simulink model "advanced_control_simulink"  (R2025b)
settings: Solver=ode3  StartTime=0.0  StopTime=50  FixedStep=0.02  RelTol=1e-3
libraries: fuzblock x1
settings Model: Creator=Mohamed Zein  LastModifiedBy=Mohamed Zein

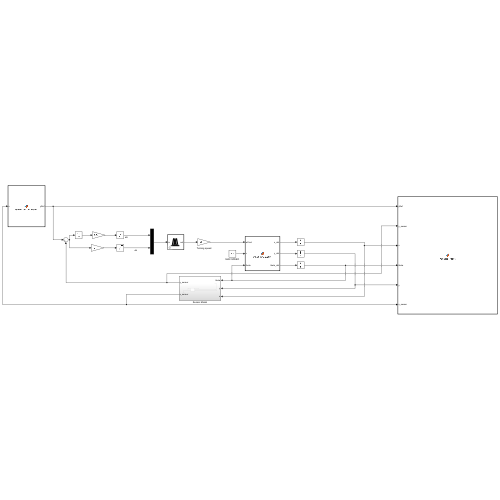
[thumbnail: Simulink's stored preview of the top-level diagram]
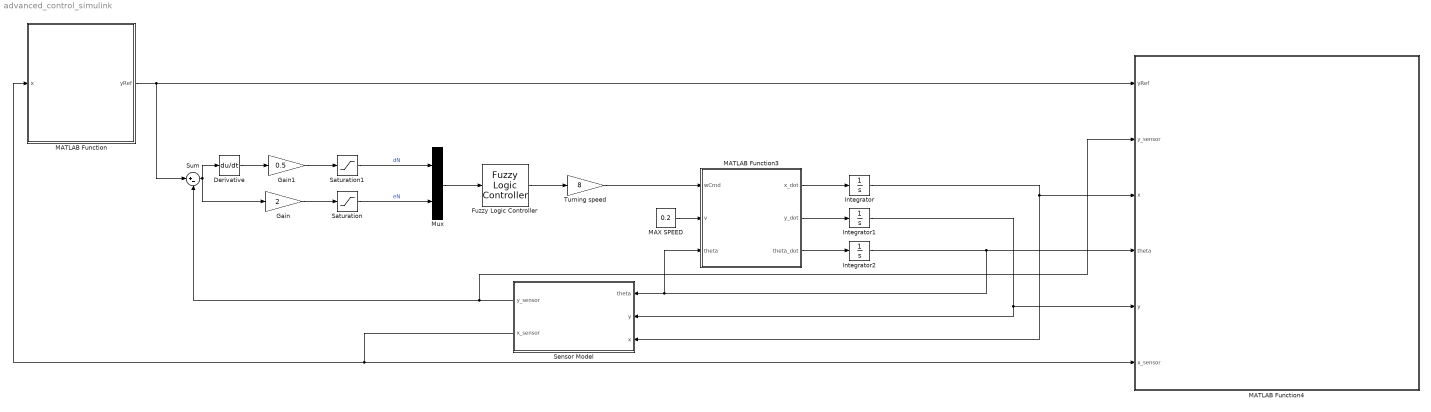
== system advanced_control_simulink ==
  Derivative : Derivative
  Fuzzy Logic Controller : fuzblock/Fuzzy Logic  Controller  FIS=fis  OutputSampleNumber=101  DataType=double  UseLookupTable=off  NumBreakpoints=10  FuzzifiedInputs=off  RuleFiringStrengths=off  RuleOutputs=off  AggregatedOutputs=off  SimulateUsing=Interpreted execution  OutOfRangeInputValueMessage=warning  NoRuleFiredMessage=warning  EmptyOutputFuzzySetMessage=warning
  Gain : Gain  Gain=2
  Gain1 : Gain  Gain=0.5
  Integrator : Integrator
  Integrator1 : Integrator  InitialCondition=1
  Integrator2 : Integrator
  MATLAB Function : MATLAB Function  TreatAsAtomicUnit=on
  MATLAB Function3 : MATLAB Function  TreatAsAtomicUnit=on
  MATLAB Function4 : MATLAB Function  TreatAsAtomicUnit=on
  MAX SPEED : Constant  Value=0.2
  Mux : Mux  Inputs=2
  Saturation : Saturate  UpperLimit=1  LowerLimit=-1
  Saturation1 : Saturate  UpperLimit=1  LowerLimit=-1
  Sensor Model : Subsystem
  Sum : Sum  Inputs=|+-
  Turning speed : Gain  Gain=8
  wires:
  MATLAB Function3/1(x_dot) -> Integrator/1
  MATLAB Function3/2(y_dot) -> Integrator1/1
  MATLAB Function3/3(theta_dot) -> Integrator2/1
  Integrator/1 -> Sensor Model/3(x), MATLAB Function4/3(x)
  MATLAB Function/1(yRef) -> Sum/1, MATLAB Function4/1(yRef)
  Turning speed/1 -> MATLAB Function3/1(wCmd)
  Integrator2/1 -> MATLAB Function3/3(theta), Sensor Model/1(theta), MATLAB Function4/4(theta)
  Integrator1/1 -> Sensor Model/2(y), MATLAB Function4/5(y)
  MAX SPEED/1 -> MATLAB Function3/2(v)
  Fuzzy Logic Controller/1 -> Turning speed/1
  Sum/1 -> Derivative/1, Gain/1
  Gain/1 -> Saturation/1
  Saturation/1 -> Mux/2  "eN"
  Gain1/1 -> Saturation1/1
  Derivative/1 -> Gain1/1
  Sensor Model/1(y_sensor) -> Sum/2, MATLAB Function4/2(y_sensor)
  Sensor Model/2(x_sensor) -> MATLAB Function/1(x), MATLAB Function4/6(x_sensor)
  Saturation1/1 -> Mux/1  "dN"
  Mux/1 -> Fuzzy Logic Controller/1

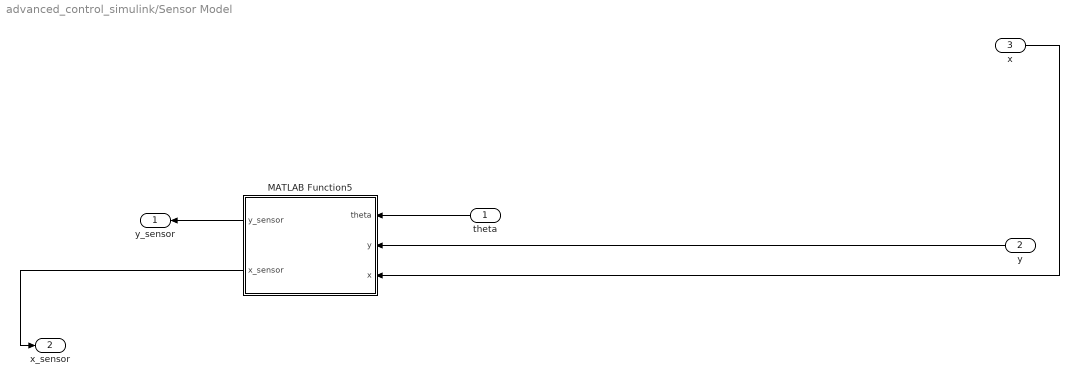
== system advanced_control_simulink/Sensor Model ==
  theta : Inport
  y : Inport  Port=2
  x : Inport  Port=3
  MATLAB Function5 : MATLAB Function  TreatAsAtomicUnit=on
  y_sensor : Outport
  x_sensor : Outport  Port=2
  wires:
  MATLAB Function5/2(x_sensor) -> x_sensor/1
  MATLAB Function5/1(y_sensor) -> y_sensor/1
  theta/1 -> MATLAB Function5/1(theta)
  x/1 -> MATLAB Function5/3(x)
  y/1 -> MATLAB Function5/2(y)

== matlab function advanced_control_simulink/MATLAB Function ==
  data: x input; yRef output
function yRef = reference_generator(x)
    % A path with sharp 90-degree corners
    if x < 1.5
        yRef = 1.0;       % Start at y = 1.0
    elseif x < 3.5
        yRef = -0.5;      % Sharp drop down to y = -0.5
    elseif x < 5.5
        yRef = 0.5;       % Sharp jump up to y = 0.5
    else
        yRef = 0.0;       % Finish at y = 0.0
    end
end

== matlab function advanced_control_simulink/MATLAB Function3 ==
  data: wCmd input; v input; theta input; x_dot output; y_dot output; theta_dot output
function [x_dot, y_dot, theta_dot] = robot_kinematics(wCmd, v, theta)
    % The integrators outside will convert these velocities into position
    theta_dot = wCmd;
    x_dot = v * cos(theta);
    y_dot = v * sin(theta);
end

== matlab function advanced_control_simulink/MATLAB Function4 ==
  data: yRef input; y_sensor input; x input; theta input; y input; x_sensor input
function visualize_robot(yRef, y_sensor ,x, theta, y,   x_sensor)
    coder.extrinsic('figure', 'plot', 'patch', 'set', 'drawnow', 'hold', 'axis', ...
        'title', 'xlabel', 'ylabel', 'legend', 'animatedline', 'addpoints', 'xlim', 'ylim', 'grid');
    
    persistent fig bodyPatch leftWheelPatch rightWheelPatch headingLine trailLine sensorBar targetDot

    bodyLength = 0.22;   
    bodyWidth  = 0.14;    
    wheelLength = 0.09;   
    wheelWidth  = 0.03;
    sensorArrayWidth = 0.15; 

    if isempty(fig)
        fig = figure('Color', 'w', 'Name', 'Simulink Live 2D Vehicle');
        hold on;
        
        % 1. PRE-DRAW THE CORNERED REFERENCE LINE
        xLine = linspace(-0.5, 7.0, 1000);
        yLine = zeros(size(xLine));
        for i = 1:length(xLine)
            if xLine(i) < 1.5
                yLine(i) = 1.0;
            elseif xLine(i) < 3.5
                yLine(i) = -0.5;
            elseif xLine(i) < 5.5
                yLine(i) = 0.5;
            else
                yLine(i) = 0.0;
            end
        end
        plot(xLine, yLine, 'k--', 'LineWidth', 1.6);
        
        % Initialize Graphics Objects
        trailLine = animatedline('Color', [0 0.45 0.74], 'LineWidth', 2.0, 'HandleVisibility', 'off');
        bodyPatch = patch('XData', nan, 'YData', nan, 'FaceColor', [0.2 0.6 0.9], 'FaceAlpha', 0.35, 'EdgeColor', [0.1 0.25 0.45], 'LineWidth', 1.5);
        leftWheelPatch = patch('XData', nan, 'YData', nan, 'FaceColor', [0.12 0.12 0.12], 'EdgeColor', [0.05 0.05 0.05], 'LineWidth', 1.0);
        rightWheelPatch = patch('XData', nan, 'YData', nan, 'FaceColor', [0.12 0.12 0.12], 'EdgeColor', [0.05 0.05 0.05], 'LineWidth', 1.0);
        headingLine = plot([nan nan], [nan nan], 'Color', [0.85 0.33 0.1], 'LineWidth', 2.0);
        
        sensorBar = plot([nan nan], [nan nan], 'r-', 'LineWidth', 3.0);
        targetDot = plot(nan, nan, 'go', 'MarkerFaceColor', 'g', 'MarkerSize', 6);
        
        axis equal; grid on;
        xlabel('x (m)'); ylabel('y (m)');
        title('Live Robot Trajectory with Cornered Path');
        legend('Reference line', 'Robot Center', 'Sensor Range', 'Target Point', 'Location', 'best');
        xlim([-0.5 7.0]); ylim([-1.5 2.0]);
    end

    % --- Vehicle Geometry Calculations ---
    bodyLocal = [ bodyLength/2, bodyLength/2, -bodyLength/2, -bodyLength/2; bodyWidth/2, -bodyWidth/2, -bodyWidth/2, bodyWidth/2 ];
    wheelY = bodyWidth/2 + wheelWidth/2;
    wheelLocal = [ -wheelLength/2, wheelLength/2; wheelY, wheelY ];
    wheelLocalMirror = wheelLocal; wheelLocalMirror(2,:) = -wheelLocalMirror(2,:);
    headingLocal = [0, bodyLength/2; 0, 0];

    transform = [cos(theta) -sin(theta); sin(theta) cos(theta)];
    bodyPts = transform * bodyLocal + [x; y];
    leftPts = transform * wheelLocal + [x; y];
    rightPts = transform * wheelLocalMirror + [x; y];
    headingPts = transform * headingLocal + [x; y];

    % --- Sensor Range Calculations ---
    dx = (sensorArrayWidth/2) * -sin(theta); 
    dy = (sensorArrayWidth/2) * cos(theta);  
    sensorBarX = [x_sensor - dx, x_sensor + dx];
    sensorBarY = [y_sensor - dy, y_sensor + dy];

    % --- Update graphics ---
    set(bodyPatch, 'XData', bodyPts(1,:), 'YData', bodyPts(2,:));
    set(leftWheelPatch, 'XData', leftPts(1,:), 'YData', leftPts(2,:));
    set(rightWheelPatch, 'XData', rightPts(1,:), 'YData', rightPts(2,:));
    set(headingLine, 'XData', headingPts(1,:), 'YData', headingPts(2,:));
    set(sensorBar, 'XData', sensorBarX, 'YData', sensorBarY);
    set(targetDot, 'XData', x_sensor, 'YData', yRef);

    addpoints(trailLine, x, y);
    drawnow limitrate;
end

== matlab function advanced_control_simulink/Sensor Model/MATLAB Function5 ==
  data: theta input; y_sensor output; y input; x input; x_sensor output
function [y_sensor, x_sensor] = sensor_model(theta, y, x)
    % Look-ahead distance (meters from center of robot to front sensor bar)
    L_sensor = 0.15; 
    
    % Calculate the coordinates of the sensor
    x_sensor = x + L_sensor * cos(theta);
    y_sensor = y + L_sensor * sin(theta);
end
